simulink model "natural_sampling"  (R2020a)
settings: Solver=VariableStepAuto  StartTime=0.0  StopTime=10.0  RelTol=1e-3
settings Model: Creator=Riyansh  LastModifiedBy=Riyansh

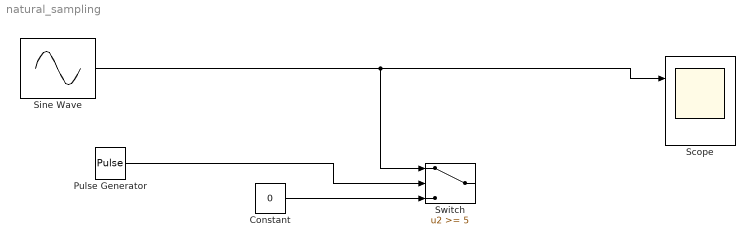
== system natural_sampling ==
  Constant : Constant  Value=0  SampleTime=1e-6
  Pulse Generator : DiscretePulseGenerator  PulseType=Time based  Amplitude=10  Period=0.01  PulseWidth=50
  Scope : Scope  NumInputPorts=2
  Sine Wave : Sin  Frequency=2*pi*5  SampleTime=1e-6
  Switch : Switch  Threshold=5
  wires:
  Sine Wave/1 -> Scope/1, Switch/1
  Constant/1 -> Switch/3
  Pulse Generator/1 -> Switch/2
